simulink model "LDRsimulink"  (R2025b)
settings: Solver=VariableStepAuto  StartTime=0.0  StopTime=10.0  MaxStep=0.01  RelTol=1e-6
settings Model: Creator=arxchy  LastModifiedBy=arxchy

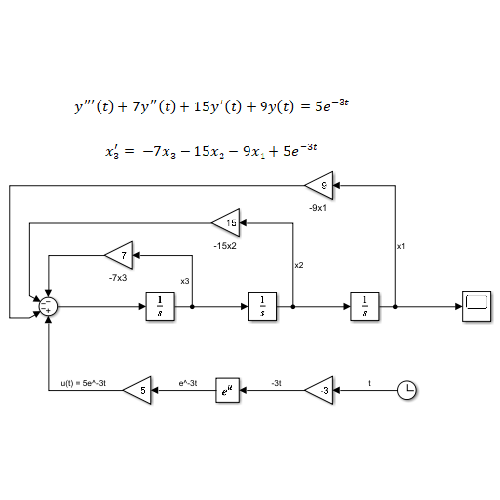
[thumbnail: Simulink's stored preview of the top-level diagram]
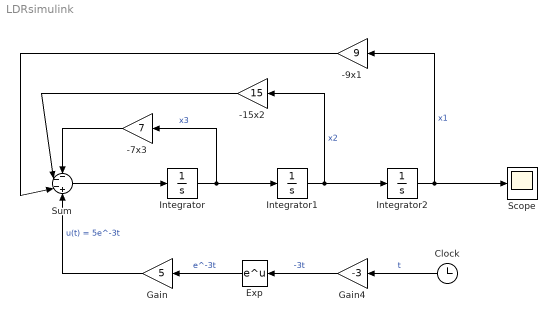
== system LDRsimulink ==
  -15x2 : Gain  Gain=15
  -7x3 : Gain  Gain=7
  -9x1 : Gain  Gain=9
  Clock : Clock
  Exp : Math
  Gain : Gain  Gain=5
  Gain4 : Gain  Gain=-3
  Integrator : Integrator  AbsoluteTolerance=1e-6
  Integrator1 : Integrator  AbsoluteTolerance=1e-6
  Integrator2 : Integrator  AbsoluteTolerance=1e-6
  Scope : Scope
      settings: ActiveDisplayYMinimum=-0.017246292180660684  ActiveDisplayYMaximum=0.095405909317226811
  Sum : Sum  Inputs=---+
  wires:
  Integrator/1 -> -7x3/1, Integrator1/1  "x3"
  Integrator1/1 -> -15x2/1, Integrator2/1  "x2"
  Integrator2/1 -> -9x1/1, Scope/1  "x1"
  Exp/1 -> Gain/1  "e^-3t"
  Gain/1 -> Sum/4  "u(t) = 5e^-3t"
  Sum/1 -> Integrator/1
  -7x3/1 -> Sum/1
  -9x1/1 -> Sum/3
  -15x2/1 -> Sum/2
  Gain4/1 -> Exp/1  "-3t"
  Clock/1 -> Gain4/1  "t"
